simulink model "untitled_restored_from_autosave"  (R2024b)
settings: Solver=VariableStepAuto  StartTime=0.0  StopTime=10.0  RelTol=1e-3
libraries: robotsim3dlib x1
settings Model: Creator=User  LastModifiedBy=User

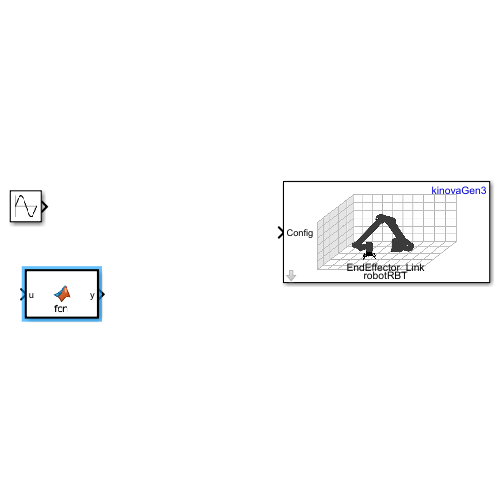
[thumbnail: Simulink's stored preview of the top-level diagram]
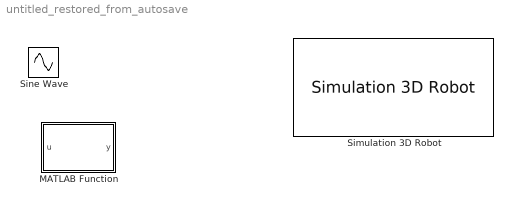
== system untitled_restored_from_autosave ==
  MATLAB Function : MATLAB Function  TreatAsAtomicUnit=on
  Simulation 3D Robot : robotsim3dlib/Simulation 3D Robot  actorInputType=Robot Library  RigidBodyTree=kinovaGen3  ActorName=robotRBT  existActorChekBox=off  initialTrans=[0 0 0]  initialRot=[0 0 0]  initialConfig="[0  0  0  0  0  0  0]"  EndEffector=EndEffector_Link  eeOffsetInpChekBox=off  eeTargetTrans=[0 0 0]  eeTargetRot=[0 0 0]  enableRegionGraspChekBox=off  regionGraspInpChekBox=off  eeTargTransDiff=[0.2 0.2 0.2]  eeTargRotDiff=[0 0 0]  inpConfEnbVal=on  inpGraspEnbVal=off  inpTransEnbVal=off  outConfEnbVal=off  outGraspEnbVal=off  outTransEnbVal=off  SampleTime=0.01  ActorType=SimulinkVehicle  ID=C  aMode=6  ActorTag=robotRBT  Mesh=RigidBodyTree
  Sine Wave : Sin  SampleTime=0

== matlab function untitled_restored_from_autosave/MATLAB Function ==
  data: u input; y output
function y = fcn(u)

y = u;
